simulink model "MATE_SynchronousMachine"  (R2024b)
settings: Solver=FixedStepDiscrete  StartTime=0.0  StopTime=6  FixedStep=Ts  RelTol=1e-4  EnableMultiTasking=on
PostLoadFcn:
  | Ts=25e-6;offset=4;
InitFcn:
  | Ts=25e-6;offset=4;
undefined symbols (not defined in the file): DiscIntNeverNeededParam, MATE, Phase, Rsnu, Single
libraries: fl_lib x79, nesl_utility x53, ee_lib x16, simetran x5, powerlib_extras x3, simulink_extras x2, simulink x2
(part 2 of 5)

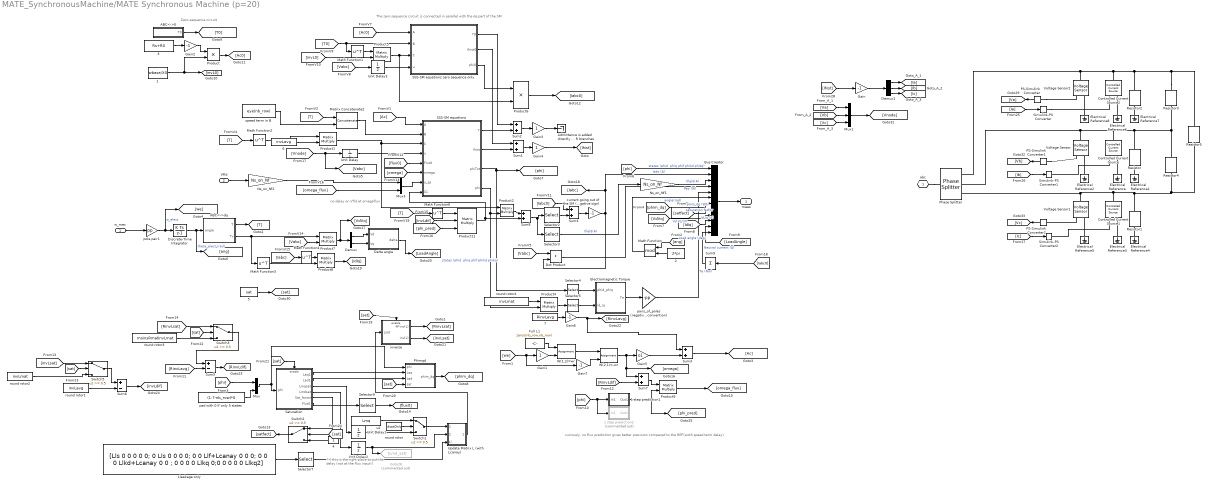
== system MATE_SynchronousMachine/MATE Synchronous Machine (p=20) ==
  note: ^
      | |
      | this is the right place to put the delay
      | (not at the flux input!)
  note: Zero-sequence circuit
  note: The zero sequence circuit is connected in parallel with the dq part of the SM
  note: curiously, no flux prediction gives better precision compared to the REF(woth speed term delay)
  note: no delay on Vfld et omegaflux
  "   w_mec" : Inport
  "   Vfld" : Inport  Port=2
  1 : Constant  Value=wbase/X0
  1 step prediction1 : Subsystem
  1 step prediction2 : Subsystem  Commented=on
  2 : Constant  Value=2*pi
  3 : Constant  Value=Rs+R0
  4 : Constant
  5 : Constant  Value=sat
  6 : Constant  Value=invLavg
  7 : Constant  Value=RinvLavg
  ABC<->0 : Subsystem
  ABC<->dq : Subsystem
  Admittance is added directly with R branches : Terminator
  Bus Creator : BusCreator  Inputs=12
  Controlled Current Source : fl_lib/Electrical/Electrical Sources/Controlled Current Source
  Controlled Current Source1 : fl_lib/Electrical/Electrical Sources/Controlled Current Source
  Controlled Current Source2 : fl_lib/Electrical/Electrical Sources/Controlled Current Source
  Delta angle : Subsystem
  Demux : Demux  Outputs=2
  Demux1 : Demux  Outputs=3
      settings: DisplayOption=none
  Discrete-Time Integrator : DiscreteIntegrator  InitialCondition=theta_0  SampleTime=Ts  ICPrevOutput=DiscIntNeverNeededParam  ICPrevScaledInput=DiscIntNeverNeededParam
  Dot Product : DotProduct  OutDataTypeStr=Inherit: Inherit via internal rule
  Electrical Reference{,1..8} (9 alike) : fl_lib/Electrical/Electrical Elements/Electrical Reference
  Electromagnetic Torque : Subsystem
  Full L1 : Constant  Value=zeros(nb_row,nb_row)
  Gain : Gain  Gain=-1
  Gain1 : Gain  SaturateOnIntegerOverflow=on  OutDataTypeStr=Inherit: Same as input  ParamDataTypeStr=Inherit: Same as input
  Gain2 : Gain  Gain=-1
  Gain3 : Gain
  Gain4 : Gain
  Gain5 : Gain  Gain=o1
  Gain6 : Gain  Gain=-1
  Gain7 : Gain  Gain=-1  SaturateOnIntegerOverflow=on  OutDataTypeStr=Inherit: Same as input  ParamDataTypeStr=Inherit: Same as input
  Goto28 : Goto  Commented=on  GotoTag=Lmd_sat
  Lleakage only : Constant  Value="[Lls 0 0 0 0 0; 0 Lls 0 0  0 0; 0 0 Llf+Lcanay 0 0 0; 0 0 0 Llkd+Lcanay 0 0 ; 0 0 0 0 Llkq 0;0 0 0 0 0 Llkq2]"
  Math Function : Math  Operator=mod  SignedPower=on
  Math Function{1..4,6} (5 alike) : Math  Operator=transpose  SignedPower=on
  Matrix Concatenate2 : Concatenate  Mode=Multidimensional array  ConcatenateDimension=2
  Mux : Mux  Inputs=2
  Mux1 : Mux  Inputs=3
  Mux3 : Mux  Inputs=2
  Ns_on_Nf1 : Gain  Gain=Ns_on_Nf
  Ns_on_Nf2 : Gain  Gain=Ns_on_Nf
  PS-Simulink Converter : nesl_utility/PS-Simulink Converter  PhysicalDomain=network_engine_domain  SubClassName=ps_output  LeftPortType=input  RightPortType=output  PseudoPeriodic=off  Frequencies=[]  VectorFormat=inherit  Unit=inherit  AffineConversion=off
  PS-Simulink Converter1 : nesl_utility/PS-Simulink Converter  PhysicalDomain=network_engine_domain  SubClassName=ps_output  LeftPortType=input  RightPortType=output  PseudoPeriodic=off  Frequencies=[]  VectorFormat=inherit  Unit=inherit  AffineConversion=off
  PS-Simulink Converter2 : nesl_utility/PS-Simulink Converter  PhysicalDomain=network_engine_domain  SubClassName=ps_output  LeftPortType=input  RightPortType=output  PseudoPeriodic=off  Frequencies=[]  VectorFormat=inherit  Unit=inherit  AffineConversion=off
  Phase Splitter : ee_lib/Connectors & References/Phase Splitter
  Phimqd : Subsystem
  Product : Product  RndMeth=Zero
  Product{1..2,4..5,7..9} (7 alike) : Product  Multiplication=Matrix(*)  SaturateOnIntegerOverflow=on  OutDataTypeStr=Inherit: Same as first input
  Product11 : Product  Inputs=3  Multiplication=Matrix(*)  SaturateOnIntegerOverflow=on  OutDataTypeStr=Inherit: Same as first input
  Product6 : Product  SaturateOnIntegerOverflow=on  OutDataTypeStr=Inherit: Same as first input
  Resistor : fl_lib/Electrical/Electrical Elements/Resistor  R=ResistanceM(2,2) Ohm  i_specify=off  i_priority=None  i=0 A  i_nominal_specify=off  i_nominal_value=1  i_nominal_unit=A  v_specify=off  v_priority=None  v=0 V  v_nominal_specify=off  v_nominal_value=1  v_nominal_unit=V
  Resistor1 : fl_lib/Electrical/Electrical Elements/Resistor  R=ResistanceM(3,3) Ohm  i_specify=off  i_priority=None  i=0 A  i_nominal_specify=off  i_nominal_value=1  i_nominal_unit=A  v_specify=off  v_priority=None  v=0 V  v_nominal_specify=off  v_nominal_value=1  v_nominal_unit=V
  Resistor2 : fl_lib/Electrical/Electrical Elements/Resistor  R=ResistanceM(1,1) Ohm  i_specify=off  i_priority=None  i=0 A  i_nominal_specify=off  i_nominal_value=1  i_nominal_unit=A  v_specify=off  v_priority=None  v=0 V  v_nominal_specify=off  v_nominal_value=1  v_nominal_unit=V
  Resistor3 : fl_lib/Electrical/Electrical Elements/Resistor  R=ResistanceM(1,2) Ohm  i_specify=off  i_priority=None  i=0 A  i_nominal_specify=off  i_nominal_value=1  i_nominal_unit=A  v_specify=off  v_priority=None  v=0 V  v_nominal_specify=off  v_nominal_value=1  v_nominal_unit=V
  Resistor4 : fl_lib/Electrical/Electrical Elements/Resistor  R=ResistanceM(2,3) Ohm  i_specify=off  i_priority=None  i=0 A  i_nominal_specify=off  i_nominal_value=1  i_nominal_unit=A  v_specify=off  v_priority=None  v=0 V  v_nominal_specify=off  v_nominal_value=1  v_nominal_unit=V
  Resistor5 : fl_lib/Electrical/Electrical Elements/Resistor  R=ResistanceM(1,3) Ohm  i_specify=off  i_priority=None  i=0 A  i_nominal_specify=off  i_nominal_value=1  i_nominal_unit=A  v_specify=off  v_priority=None  v=0 V  v_nominal_specify=off  v_nominal_value=1  v_nominal_unit=V
  SSS-SM equations : Subsystem
  SSS-SM equations zero sequence only : Subsystem
  Saturation : Subsystem
  Selector2 : Selector  InputPortWidth=4  IndexOptions=Index vector (dialog)  Indices=[1 2 3 ]  OutputSizes=1
  Selector3 : Selector  InputPortWidth=4  IndexOptions=Index vector (dialog)  Indices=[4 ]  OutputSizes=1
  Selector4 : Selector  InputPortWidth=nb_row  IndexOptions=Index vector (dialog)  Indices=[1 2]  OutputSizes=1
  Selector5 : Selector  InputPortWidth=nb_row  IndexOptions=Index vector (dialog)  Indices=[1 2]  OutputSizes=1
  Selector7 : Selector  NumberOfDimensions=2  InputPortWidth=3  IndexOptions=Index vector (dialog),Index vector (dialog)  Indices=[1:nb_row],[1:nb_row]  OutputSizes=1,1
  Selector9 : Selector  InputPortWidth=6  IndexOptions=Index vector (dialog)  Indices=[1:nb_row]  OutputSizes=1
  Simulink-PS Converter : nesl_utility/Simulink-PS Converter  PhysicalDomain=network_engine_domain  SubClassName=ps_input  LeftPortType=input  RightPortType=output  PseudoPeriodic=off  Frequencies=[]  NoiseDistribution=none  NoiseParameters=[]  Unit=1  AffineConversion=off  FilteringAndDerivatives=provide  SimscapeFilterOrder=1  InputFilterTimeConstant=0.001  UdotUserProvided=0
  Simulink-PS Converter1 : nesl_utility/Simulink-PS Converter  PhysicalDomain=network_engine_domain  SubClassName=ps_input  LeftPortType=input  RightPortType=output  PseudoPeriodic=off  Frequencies=[]  NoiseDistribution=none  NoiseParameters=[]  Unit=1  AffineConversion=off  FilteringAndDerivatives=provide  SimscapeFilterOrder=1  InputFilterTimeConstant=0.001  UdotUserProvided=0
  Simulink-PS Converter2 : nesl_utility/Simulink-PS Converter  PhysicalDomain=network_engine_domain  SubClassName=ps_input  LeftPortType=input  RightPortType=output  PseudoPeriodic=off  Frequencies=[]  NoiseDistribution=none  NoiseParameters=[]  Unit=1  AffineConversion=off  FilteringAndDerivatives=provide  SimscapeFilterOrder=1  InputFilterTimeConstant=0.001  UdotUserProvided=0
  Sum{1..4,7..8} (6 alike) : Sum  SaturateOnIntegerOverflow=on
  Sum5 : Sum  Inputs=+-  SaturateOnIntegerOverflow=on
  Sum6 : Sum  Inputs=+-  SaturateOnIntegerOverflow=on
  Sum9 : Sum  Inputs=+  SaturateOnIntegerOverflow=on
  Switch{1..3,5} (4 alike) : Switch  Threshold=0.5  SaturateOnIntegerOverflow=off  InputSameDT=off
  Unit Delay : UnitDelay  SampleTime=Ts  HasFrameUpgradeWarning=on
  Unit Delay1 : UnitDelay  InitialCondition=Lmq  SampleTime=Ts  HasFrameUpgradeWarning=on
  Unit Delay2 : UnitDelay  InitialCondition=Lmd  SampleTime=Ts  HasFrameUpgradeWarning=on
  Unit Delay3 : UnitDelay  SampleTime=Ts  HasFrameUpgradeWarning=on
  Update Matrix L (with Lcanay) : Subsystem
  Voltage Sensor : fl_lib/Electrical/Electrical Sensors/Voltage Sensor
  Voltage Sensor1 : fl_lib/Electrical/Electrical Sensors/Voltage Sensor
  Voltage Sensor2 : fl_lib/Electrical/Electrical Sensors/Voltage Sensor
  W(1,2)=wr : Assignment  NumberOfDimensions=2  IndexOptions=Index vector (dialog),Index vector (dialog)  Indices=1,2  OutputSizes=1,1
  W(2,1)=-wr : Assignment  NumberOfDimensions=2  IndexOptions=Index vector (dialog),Index vector (dialog)  Indices=2,1  OutputSizes=1,1
  current going out of the SM (negative sign) : Gain  Gain=-1
  inverse : Subsystem
  pad with 0 if only 5 states : Constant  Value=(1:7-nb_row)*0
  pairs_of_poles (negative sign for generator convention) : Gain  Gain=-pp
  pole pair1 : Gain  Gain=pp
  round rotor : Constant  Value=dsatOnly
  round rotor1 : Constant  Value=invLavg
  round rotor2 : Constant  Value=invLmat
  round rotor3 : Constant  Value=moinsRmatinvLmat
  round rotor4 : Constant  Value=invLmat
  speed term in B : Constant  Value=eye(nb_row)  VectorParams1D=off
  u2 : Constant  Value=Lmq
  "abc   " : PMIOPort  Side=Right
  "meas   " : Outport
  wires:
  Mux3/1 -> SSS-SM equations/7(u_sp)
  1 step prediction1/1(Out1) -> Product9/2, [phi_pred]
  [sat] -> Switch2/2
  Switch5/1 -> Sum6/1
  [sat] -> Switch5/2
  [sat] -> Switch3/2
  [sat] -> Saturation/Enable
  [sat] -> Phimqd/4(sat)
  [sat] -> inverse/Enable
  5/1 -> [sat]
  [invLsat] -> Switch5/1
  round rotor2/1 -> Switch5/3
  inverse/2(inv(L)) -> [invLsat]
  Gain3/1 -> Admittance is added directly with R branches/1
  "   Vfld"/1 -> Ns_on_Nf2/1
  Ns_on_Nf2/1 -> Mux3/1
  Switch3/1 -> Sum5/1
  [RinvLsat] -> Switch3/1
  round rotor3/1 -> Switch3/3
  inverse/1(-R*inv(L)) -> [RinvLsat]
  Update Matrix L (with Lcanay)/1(Lsat) -> inverse/1(Lsat)
  Sum9/1 -> Bus Creator/12  "Neutral current (A)"
  [Iabc0] -> Sum9/1
  [Vnode] -> Unit Delay/1, [Vabc]
  SSS-SM equations zero sequence only/2(Ihist0) -> Sum1/1
  SSS-SM equations zero sequence only/1(Y0) -> Sum2/1
  [phi] -> 1 step prediction2/1(In1), 1 step prediction1/1(In1)
  [omega_flux] -> Mux3/2
  round rotor4/1 -> Product4/1
  Product11/1 -> Sum8/2, SSS-SM equations/8(C1)
  Sum8/1 -> Selector2/1, Selector3/1
  Product2/1 -> Sum8/1
  [Iabc0] -> Sum4/1
  [phi_pred] -> Product11/3
  [invLdif] -> Product11/2
  Math Function6/1 -> Product11/1
  [T] -> Math Function6/1
  Sum6/1 -> [invLdif]
  round rotor1/1 -> Sum6/2
  6/1 -> Product1/2
  Sum7/1 -> Product9/1
  [RinvLdif] -> Sum7/2
  Sum5/1 -> [RinvLdif]
  Gain6/1 -> [RinvLavg], Sum3/1
  [RinvLavg] -> Sum5/2
  7/1 -> Gain6/1
  Ns_on_Nf1/1 -> Bus Creator/3  "Ifield(A)"
  Product9/1 -> [omega_flux]
  Bus Creator/1 -> "meas   "/1
  Matrix Concatenate2/1 -> SSS-SM equations/2(B)
  speed term in B/1 -> Matrix Concatenate2/2
  [T] -> Matrix Concatenate2/1
  Gain5/1 -> Sum3/2
  ABC<->dq/2(Tv) -> Product7/1, Math Function3/1
  [LoadAngle] -> Bus Creator/11  "Load angle (deg)"
  [IdIq] -> Bus Creator/10  "Id Iq (A)"
  [VdVq] -> Bus Creator/9  "Vd Vq (V)"
  Math Function4/1 -> Product8/1
  Math Function3/1 -> Product8/2
  [Iabc] -> Math Function4/1
  Product8/1 -> [IdIq]
  Delta angle/1(delta) -> [LoadAngle]
  [Vabc] -> Product7/2
  Demux/1 -> Delta angle/1(Vd)
  Demux/2 -> Delta angle/2(Vq)
  Product7/1 -> Demux/1, [VdVq]
  pole pair1/1 -> [we], Discrete-Time Integrator/1  "w_elect"
  ABC<->dq/1(T) -> [T]
  Discrete-Time Integrator/1 -> ABC<->dq/1(angle), [ang]  "theta_elect (rad)"
  SSS-SM equations/3(phiTot) -> [phi], Selector4/1  "states (phid  phiq phif phikd phikq)"
  Unit Delay/1 -> SSS-SM equations/4(u)
  Gain7/1 -> W(2,1)=-wr/2
  W(1,2)=wr/1 -> W(2,1)=-wr/1
  [we] -> Gain1/1, Gain7/1
  [T] -> Math Function2/1
  Product1/1 -> Product2/1, SSS-SM equations/3(C)
  Math Function2/1 -> Product1/1
  Gain1/1 -> W(1,2)=wr/2
  Selector3/1 -> Ns_on_Nf1/1  "Ifield(A)"
  Electromagnetic Torque/1(Te) -> pairs_of_poles (negative sign for generator convention)/1
  Selector5/1 -> Electromagnetic Torque/2(id_iq)
  Selector4/1 -> Electromagnetic Torque/1(phid_phiq)
  Product4/1 -> Selector5/1
  pairs_of_poles (negative sign for generator convention)/1 -> Bus Creator/5  "Te (Nm)"
  [Vabc] -> Dot Product/1
  Dot Product/1 -> Bus Creator/4  "Peo (W)"
  current going out of the SM (negative sign)/1 -> [Iabc], Bus Creator/2, Dot Product/2  "Iabc (A)"
  "   w_mec"/1 -> pole pair1/1
  [ang] -> Math Function/1
  Math Function/1 -> Bus Creator/6  "angle(rad)"
  2/1 -> Math Function/2
  [phi] -> Mux/1
  Saturation/1(Laq1) -> Phimqd/2(Laq)
  Saturation/2(Lad1) -> Phimqd/3(Lad)
  Saturation/3(Lmqsat) -> Unit Delay1/1
  Saturation/4(Lmdsat) -> Unit Delay2/1
  Switch1/1 -> Update Matrix L (with Lcanay)/1(Lmq)
  round rotor/1 -> Switch1/2
  Unit Delay2/1 -> Goto28/1, Update Matrix L (with Lcanay)/2(Lmd)
  Lleakage only/1 -> Selector7/1
  [phim_dq] -> Bus Creator/7  "phim_dq (Wb)"
  Phimqd/1(phim_dq) -> [phim_dq]
  Unit Delay1/1 -> Switch1/3
  u2/1 -> Switch1/1
  Selector7/1 -> Update Matrix L (with Lcanay)/3(Ll)
  [Ac] -> SSS-SM equations/1(A)
  pad with 0 if only 5 states/1 -> Mux/2
  Mux/1 -> Saturation/1(phi), Phimqd/1(phi)
  ABC<->0/1(T0) -> [T0]
  3/1 -> Gain2/1
  Gain2/1 -> Product/1
  1/1 -> [invL0], Product/2
  Product/1 -> [Ac0]
  [Ac0] -> SSS-SM equations zero sequence only/1(A)
  [Vabc] -> Unit Delay3/1
  Unit Delay3/1 -> SSS-SM equations zero sequence only/4(u)
  [T0] -> Math Function1/1, SSS-SM equations zero sequence only/2(B)
  Math Function1/1 -> Product5/1
  [invL0] -> Product5/2
  Product5/1 -> Product6/2, SSS-SM equations zero sequence only/3(C)
  Sum1/1 -> Gain4/1
  SSS-SM equations/2(Ihist) -> Sum1/2
  SSS-SM equations/1(Y) -> Sum2/2
  Sum2/1 -> Gain3/1
  Selector2/1 -> Sum4/2
  Sum4/1 -> current going out of the SM (negative sign)/1
  [satfact] -> Bus Creator/8  "saturation factor"
  Switch2/1 -> [satfact]
  Saturation/5(Sat_factor) -> Switch2/1
  4/1 -> Switch2/3
  Saturation/6(Flux0) -> Selector9/1
  [flux0] -> SSS-SM equations/5(Flux0)
  W(2,1)=-wr/1 -> [omega], Sum7/1, Gain5/1
  Sum3/1 -> [Ac]
  Full L1/1 -> W(1,2)=wr/1
  [omega] -> SSS-SM equations/6(omega)
  [phi] -> Bus Creator/1  "states (phid  phiq phif phikd phikq)"
  Selector9/1 -> [flux0]
  SSS-SM equations/4(phi) -> Product2/2, Product4/2
  PS-Simulink Converter1/1 -> [Vb]
  Mux1/1 -> [Vnode]
  Demux1/2 -> [Ib]
  Demux1/1 -> [Ia]
  [Vc] -> Mux1/3
  Gain/1 -> Demux1/1
  PS-Simulink Converter/1 -> [Va]
  [Ic] -> Simulink-PS Converter2/1
  Demux1/3 -> [Ic]
  [Va] -> Mux1/1
  [Ihist] -> Gain/1
  [Vb] -> Mux1/2
  PS-Simulink Converter2/1 -> [Vc]
  [Ib] -> Simulink-PS Converter1/1
  [Ia] -> Simulink-PS Converter/1
  Gain4/1 -> [Ihist]
  SSS-SM equations zero sequence only/3(phi0) -> Product6/1
  Product6/1 -> [Iabc0]
  connections:
  Controlled Current Source/LConn1 -- Resistor4/LConn1 -- Resistor3/RConn1 -- Resistor/LConn1 -- Phase Splitter/RConn2 -- Voltage Sensor/LConn1
  Resistor4/RConn1 -- Resistor5/RConn1 -- Controlled Current Source1/LConn1 -- Phase Splitter/RConn3 -- Voltage Sensor1/LConn1 -- Resistor1/LConn1
  Resistor3/LConn1 -- Resistor5/LConn1 -- Resistor2/LConn1 -- Controlled Current Source2/LConn1 -- Phase Splitter/RConn1 -- Voltage Sensor2/LConn1
  Electrical Reference2/LConn1 -- Voltage Sensor/RConn2
  Electrical Reference3/LConn1 -- Controlled Current Source1/RConn2
  Electrical Reference1/LConn1 -- Resistor/RConn1
  Electrical Reference7/LConn1 -- Resistor2/RConn1
  Controlled Current Source1/RConn1 -- Simulink-PS Converter2/RConn1
  "abc   "/RConn1 -- Phase Splitter/LConn1
  Electrical Reference4/LConn1 -- Resistor1/RConn1
  Electrical Reference6/LConn1 -- Controlled Current Source2/RConn2
  PS-Simulink Converter1/LConn1 -- Voltage Sensor/RConn1
  Simulink-PS Converter/RConn1 -- Controlled Current Source2/RConn1
  Electrical Reference/LConn1 -- Controlled Current Source/RConn2
  Voltage Sensor1/RConn1 -- PS-Simulink Converter2/LConn1
  Controlled Current Source/RConn1 -- Simulink-PS Converter1/RConn1
  PS-Simulink Converter/LConn1 -- Voltage Sensor2/RConn1
  Electrical Reference8/LConn1 -- Voltage Sensor2/RConn2
  Electrical Reference5/LConn1 -- Voltage Sensor1/RConn2

== system MATE_SynchronousMachine/MATE_LineCommutatedConverter ==
  g : Inport
  MATEPREP : Subsystem  Commented=on
  MATE_AGGREG : Subsystem
  Phase Splitter2 : ee_lib/Connectors & References/Phase Splitter
  abc : PMIOPort  Side=Left
  + : PMIOPort  Port=2  Side=Right
  - : PMIOPort  Port=3  Side=Right
  meas : Outport
  wires:
  g/1 -> MATEPREP/1(g), MATE_AGGREG/1(g)
  MATE_AGGREG/1(meas) -> meas/1
  connections:
  MATEPREP/RConn2 -- MATE_AGGREG/RConn2 -- -/RConn1
  MATEPREP/RConn1 -- MATE_AGGREG/RConn1 -- +/RConn1
  Phase Splitter2/RConn1 -- MATEPREP/LConn1 -- MATE_AGGREG/LConn1
  Phase Splitter2/RConn2 -- MATEPREP/LConn2 -- MATE_AGGREG/LConn2
  Phase Splitter2/RConn3 -- MATEPREP/LConn3 -- MATE_AGGREG/LConn3
  abc/RConn1 -- Phase Splitter2/LConn1

== system MATE_SynchronousMachine/Mesure et visualisation ==
  Discrete Mean value : Subsystem  mask(Discrete Mean value){Freq=60, Vinit=0, Ts=Ts}
      mask prompts: Freq "Fundamental frequency (Hz):"; Vinit "Initial input (DC component):"; Ts "Sample time:"
      mask help: Compute the mean value of the input signal over a running window of one cycle of the specified fundamental frequency.
      mask init:
      | SamplesPerCycle=1/Freq/Ts;
      | RoundSamplesPerCycle=ceil(SamplesPerCycle);
      | Delay=RoundSamplesPerCycle*Ts;
      | Corr1=(SamplesPerCycle-RoundSamplesPerCycle)/2;
      | Corr2=(SamplesPerCycle-RoundSamplesPerCycle)/SamplesPerCycle;
      | K1=Corr1*Corr2;
      | K2=Corr2 + Corr1*Corr2;
      mask Display: disp('Mean\n(discrete)')
  Mux : Mux  Inputs=2
  Mux3 : Mux  Inputs=2
  Mux4 : Mux  Inputs=2
  V1 Vref : Outport
  If IIfref : Outport  Port=2
  Vcc : Outport  Port=3
  wires:
  Discrete Mean value/1(Mean) -> Mux/2
  [Ucc] -> Mux/1, Discrete Mean value/1(In)
  Mux/1 -> Vcc/1  "Vcc - Vcc moyen (V)"
  [If] -> Mux3/1
  [Ifref] -> Mux3/2
  Mux3/1 -> If IIfref/1
  [V1] -> Mux4/1
  [Vref] -> Mux4/2
  Mux4/1 -> V1 Vref/1

== system MATE_SynchronousMachine/Model Initialization ==

== system MATE_SynchronousMachine/PQ ==
  note: 1) P = Va*Ia + Vb*Ib + Vc*Ic
  note: 2) Q = 1/sqrt(3)* (Vbc*Ia + Vca*Ib + Vab*Ic)
  note: This block computes the 3-phase instantaneous real power and reactive power using the following equations:
  note: Note: Equation 2 is valid only for a balanced and harmonic-free system.
  Vabc : Inport  PortDimensions=3
  Iabc : Inport  Port=2  PortDimensions=3
  Demux : Demux  Outputs=3
      settings: DisplayOption=none
  Mux : Mux  Inputs=3
  Mux1 : Mux  Inputs=2
  Product1 : Product  InputSameDT=on  SaturateOnIntegerOverflow=on  OutDataTypeStr=Inherit: Same as first input
  Product3 : Product  InputSameDT=on  SaturateOnIntegerOverflow=on  OutDataTypeStr=Inherit: Same as first input
  Sum : Sum  Inputs=+-  InputSameDT=on  SaturateOnIntegerOverflow=on  OutDataTypeStr=Inherit: Same as first input
  Sum1 : Sum  Inputs=1  InputSameDT=on  SaturateOnIntegerOverflow=on  OutDataTypeStr=Inherit: Same as first input
  Sum4 : Sum  Inputs=1  InputSameDT=on  SaturateOnIntegerOverflow=on  OutDataTypeStr=Inherit: Same as first input
  Sum5 : Sum  Inputs=+-  InputSameDT=on  SaturateOnIntegerOverflow=on  OutDataTypeStr=Inherit: Same as first input
  Sum6 : Sum  Inputs=+-  InputSameDT=on  SaturateOnIntegerOverflow=on  OutDataTypeStr=Inherit: Same as first input
  pu->V : Gain  Gain=1/sqrt(3)  SaturateOnIntegerOverflow=on  OutDataTypeStr=Inherit: Same as input  ParamDataTypeStr=Inherit: Same as input
  PQ : Outport  VectorParamsAs1DForOutWhenUnconnected=off
  wires:
  Sum1/1 -> pu->V/1
  Product3/1 -> Sum1/1
  Product1/1 -> Sum4/1
  Vabc/1 -> Product1/1, Demux/1
  Iabc/1 -> Product1/2, Product3/2
  Sum4/1 -> Mux1/1  "P"
  Demux/1 -> Sum/1, Sum6/2
  Demux/2 -> Sum/2, Sum5/1
  Demux/3 -> Sum5/2, Sum6/1
  Sum/1 -> Mux/3
  Sum5/1 -> Mux/1
  Sum6/1 -> Mux/2
  Mux/1 -> Product3/1
  pu->V/1 -> Mux1/2  "Q"
  Mux1/1 -> PQ/1

== system MATE_SynchronousMachine/VI meas ==
  Kv2 : Gain  Gain=Kv  SaturateOnIntegerOverflow=on  OutDataTypeStr=Inherit: Same as input  ParamDataTypeStr=Inherit: Same as input
  Kv3 : Gain  Gain=Ki  SaturateOnIntegerOverflow=on  OutDataTypeStr=Inherit: Same as input  ParamDataTypeStr=Inherit: Same as input
  Meas : ee_lib/Sensors & Transducers/Current and Voltage Sensor (Three-Phase)  vMeasurementType=ee.enum.vmeasurement.lg  outputUnit=ee.enum.unit.si  SRated=100e6 A*V  VRated=24e3 V  I_specify=off  I_priority=None  I=[0, 0, 0] A  I_nominal_specify=off  I_nominal_value=1  I_nominal_unit=A  V_specify=off  V_priority=None  V=[0, 0, 0] V  V_nominal_specify=off  V_nominal_value=1  V_nominal_unit=V
      settings: InternalSimscapePortConfiguration="{\"Bottom\":[],\"Left\":[{\"id\":\"N1\",\"label\":\"~1\",\"type\":\"foundation.electrical.three_phase\"}],\"Right\":[{\"id\":\"V_output\",\"label\":\"V\",\"type\":\"output\"},{\"id\":\"I_output\",\"label\":\"I\",\"type\":\"output\"},{\"id\":\"N2\",\"label\":\"~2\",\"type\":\"foundation.electrical.three_phase\"}],\"Top\":[]}"
  PS-Simulink Converter : nesl_utility/PS-Simulink Converter  PhysicalDomain=network_engine_domain  SubClassName=ps_output  LeftPortType=input  RightPortType=output  PseudoPeriodic=off  Frequencies=[]  VectorFormat=inherit  Unit=inherit  AffineConversion=off
  PS-Simulink Converter1 : nesl_utility/PS-Simulink Converter  PhysicalDomain=network_engine_domain  SubClassName=ps_output  LeftPortType=input  RightPortType=output  PseudoPeriodic=off  Frequencies=[]  VectorFormat=inherit  Unit=inherit  AffineConversion=off
  + : PMIOPort  Side=Left
  - : PMIOPort  Port=2  Side=Right
  tag scope: IabcB13_8=global, VabcB13_8=global
  wires:
  Kv3/1 -> [IabcB13_8]
  Kv2/1 -> [VabcB13_8]
  PS-Simulink Converter1/1 -> Kv3/1
  PS-Simulink Converter/1 -> Kv2/1
  connections:
  Meas/RConn1 -- PS-Simulink Converter/LConn1
  Meas/LConn1 -- +/RConn1
  Meas/RConn2 -- PS-Simulink Converter1/LConn1
  Meas/RConn3 -- -/RConn1

== system MATE_SynchronousMachine/VI meas1 ==
  Kv2 : Gain  Gain=Kv  SaturateOnIntegerOverflow=on  OutDataTypeStr=Inherit: Same as input  ParamDataTypeStr=Inherit: Same as input
  Kv3 : Gain  Gain=Ki  SaturateOnIntegerOverflow=on  OutDataTypeStr=Inherit: Same as input  ParamDataTypeStr=Inherit: Same as input
  Meas : ee_lib/Sensors & Transducers/Current and Voltage Sensor (Three-Phase)  vMeasurementType=ee.enum.vmeasurement.lg  outputUnit=ee.enum.unit.si  SRated=100e6 A*V  VRated=24e3 V  I_specify=off  I_priority=None  I=[0, 0, 0] A  I_nominal_specify=off  I_nominal_value=1  I_nominal_unit=A  V_specify=off  V_priority=None  V=[0, 0, 0] V  V_nominal_specify=off  V_nominal_value=1  V_nominal_unit=V
      settings: InternalSimscapePortConfiguration="{\"Bottom\":[],\"Left\":[{\"id\":\"N1\",\"label\":\"~1\",\"type\":\"foundation.electrical.three_phase\"}],\"Right\":[{\"id\":\"V_output\",\"label\":\"V\",\"type\":\"output\"},{\"id\":\"I_output\",\"label\":\"I\",\"type\":\"output\"},{\"id\":\"N2\",\"label\":\"~2\",\"type\":\"foundation.electrical.three_phase\"}],\"Top\":[]}"
  PS-Simulink Converter : nesl_utility/PS-Simulink Converter  PhysicalDomain=network_engine_domain  SubClassName=ps_output  LeftPortType=input  RightPortType=output  PseudoPeriodic=off  Frequencies=[]  VectorFormat=inherit  Unit=inherit  AffineConversion=off
  PS-Simulink Converter1 : nesl_utility/PS-Simulink Converter  PhysicalDomain=network_engine_domain  SubClassName=ps_output  LeftPortType=input  RightPortType=output  PseudoPeriodic=off  Frequencies=[]  VectorFormat=inherit  Unit=inherit  AffineConversion=off
  + : PMIOPort  Side=Left
  - : PMIOPort  Port=2  Side=Right
  tag scope: Ifault=global, Vfault=global
  wires:
  PS-Simulink Converter/1 -> Kv2/1
  PS-Simulink Converter1/1 -> Kv3/1
  Kv2/1 -> [Vfault]
  Kv3/1 -> [Ifault]
  connections:
  Meas/RConn3 -- -/RConn1
  Meas/RConn2 -- PS-Simulink Converter1/LConn1
  Meas/LConn1 -- +/RConn1
  Meas/RConn1 -- PS-Simulink Converter/LConn1

== system MATE_SynchronousMachine/turbine1 ==
  feild : Inport
  Te : Inport  Port=2
  Peo : Inport  Port=3
  Gain : Gain  Gain=1/(2*pi*60/20)
  Gain1 : Gain  Gain=1/202e6
  Gain3 : Gain  Gain=202e6
  Gain4 : Gain  Gain=1/(2*pi*60/20)
  Hydraulic Turbine and Governor : Subsystem  mask(Hydraulic Turbine and Governor){sm=[ 10/3  0.07 ], gate=[  0.01  0.97518  -0.1  0.1 ], reg=[  0.05  1.163  0.105  0  0.01  ], hyd=[  0  2.67  ], dref=0, po=0.802}
      mask prompts: sm "Servo-motor [ Ka()  Ta(sec) ]:"; gate "Gate opening limits [ gmin,gmax(pu)    vgmin,vgmax(pu/s) ]:"; reg "Permanent droop and regulator  [ Rp() Kp() Ki() Kd() Td(s) ]:"; hyd "Hydraulic turbine [ beta()  Tw(sec) ]:"; dref "Droop reference (0=power error, 1=gate opening):"; po "Initial mechanical power (pu):"
      mask help: Implements a hydraulic turbine combined to a PID governor system.
      mask init:
      | %block = gcb;
      | %[Ts, WantBlockChoice,ka,ta,gmin,gmax,vgmin,vgmax,Rp,Kp,ki,kd,td,beta,tw,go] = powericon('HydraulicTurbineInit',block,sm,gate,reg,hyd,po);
      | ka =sm (1 ); 
      | ta =sm (2 ); 
      | gmin =gate (1 ); 
      | gmax =gate (2 ); 
      | vgmin =gate (3 ); 
      | vgmax =gate (4 ); 
      | Rp =reg (1 ); 
      | kp =reg (2 ); 
      | ki =reg (3 ); 
      | kd =reg (4 ); 
      | td =reg (5 ); 
      | beta =hyd (1 ); 
      | tw =hyd (2 ); 
      | go =po *(gmax -gmin ); 
      | %powericon('SetInternalModels','set',block,WantBlockChoice);
      settings: OpenFcn=sps_rtmsupport('OpenFcn',gcbh)
      mask Help: helpview(psbhelp);
      mask Display: disp('')
  Mechanical model : Subsystem  mask(Synchronous machine mechanical model){J=3.4111e+06, F=0, fo=60/20, Ts=Ts}
      mask prompts: J "Inertia (kg.m^2)"; F "Friction (N.n.s)"; fo "Initial mechanical frequency (Hz)"; Ts "Sample Time (s)"
      mask help:
      | This is the mechanical equation of a synchronous machine.
      |
      | all values in SI.
      | J: inertia
      | F:friction
      | Te: torque input from the SM
      | Pin: power from the turbine
      | wmec: mechanical speed of the SM.
      | delta_wm: speed deviation
  Pref : Constant  Value=0.8
  Product1 : Product
  Terminator : Terminator
  wref : Constant
  w : Outport
  wires:
  Hydraulic Turbine and Governor/2(gate) -> Terminator/1
  Hydraulic Turbine and Governor/1(Pm) -> Gain3/1
  Gain1/1 -> Hydraulic Turbine and Governor/4(Pe0)
  Gain/1 -> Hydraulic Turbine and Governor/3(we)
  wref/1 -> Hydraulic Turbine and Governor/1(wref)
  Mechanical model/2(delta_wm) -> Gain4/1
  Pref/1 -> Product1/2
  Product1/1 -> Hydraulic Turbine and Governor/2(Pref)
  Gain3/1 -> Mechanical model/2(Pin)
  Mechanical model/1(wmec) -> Gain/1, w/1
  Gain4/1 -> Hydraulic Turbine and Governor/5(dw)
  feild/1 -> Product1/1
  Te/1 -> Mechanical model/1(Te)
  Peo/1 -> Gain1/1

== system MATE_SynchronousMachine/Command/Regulateur de courant ==
  If (pu) : Inport
  If_ref : Inport  Port=2
  Discrete 1st-Order Filter : Subsystem  mask(Discrete 1st-Order Filter){FilterType=Lowpass, Tc=1e-3, Ts=Ts, Initialize=off, Vac_Init=[0, 0, 60], Vdc_Init=0, PlotResponse=off, param1=[1 500 0.1]}
      mask prompts: FilterType "Filter Type:"; Tc "Time constant (s):"; Ts "Sample time:"; Initialize "Initialize filter states"; Vac_Init "AC initial input: [ Mag  Phase(degrees)  Freq(Hz) ]"; Vdc_Init "DC Initial input:"; PlotResponse "Plot filter response"; param1 "Frequency range(Hz) : [Start  End  Inc.]"
      mask init:
      | switch FilterType
      | case 1, % Lowpass
      |     X=[0 1 2 3 4];
      |     Y=[-2 -2 -3 -4 -4];
      |     numc=1;
      |     denc=[Tc 1];
      | case 2,   % Highpass
      |     X=[0 1 2 3 4];
      |     Y=[-4 -4 -3 -2 -2];
      |     numc=[1 0];
      |     denc=[1 1/Tc];
      | end
      | %
      | [Ac,Bc,Cc,Dc]=tf2ss(numc,denc);
      | %
      | %  Conversion to discrete transfer function
      | nstates = size(Ac,1);
      | if Ts<=0
      |     message = 'The Sample time parameter must be greater than zero. Note that specifying inherited sample time (-1) does not work for this block';
      |     error(message);
      | end
      | invexp = inv(eye(nstates) - (Ts/2)*Ac);
      | Ad = invexp*(eye(nstates) + (Ts/2)*Ac);
      | Bd = invexp*Bc;
      | Cd = Cc*invexp*Ts;
      | Dd = Cc*invexp*Bc*(Ts/2) + Dc;
      | %
      | if Initialize==1  % Compute initial conditions on states
      |     u1=Vac_Init(1)*exp(j*Vac_Init(2)*pi/180);
      |     u2=Vdc_Init*exp(j*90*pi/180);
      |     u=u1+u2;
      |     u0=imag(u); % input at  t=0;
      |     I=eye(size(Ac));
      |     sI1=I*j*(2*pi*Vac_Init(3));
      |     sI2=I*j*0;
      |     x=inv(sI1-Ac)*Bc*u1 + inv(sI2-Ac)*Bc*u2;
      |     x0c=imag(x);
      |     x0d=(I-Ac*Ts/2)*x0c/Ts - Bc/2*u0;
      | else
      |     x0d=0;
      | end
      | 
      | %
      | if PlotResponse==1 % Plot frequency and step response
      | t=[0:Tc/1000:7*Tc];
      | f=param1(1):param1(3):param1(2);
      | w=2*pi*f;
      | switch FilterType
      | 	case 1, % Lowpass
      | 		Ystep=1 - exp(-t/Tc);
      | 		RepFreq=1./(1+Tc*j.*w);
      | 	case 2,   % Highpass
      | 		Ystep=exp(-t/Tc);
      | 		RepFreq=1./(1 + (1./(Tc*j.*w)));
      | end
      | %
      | Mag=abs(RepFreq);
      | Pha=angle(RepFreq)*180/pi;
      | %
      | figure(1)
      | subplot(2,1,1)
      | plot(f,Mag)
      | grid
      | title('Bode Diagram')
      | ylabel('Magnitude')
      | subplot(2,1,2)
      | plot(f,Pha)
      | ylabel('Phase (deg)')
      | xlabel('Frequency (Hz)')
      | grid
      | figure(2)
      | plot(t,Ystep)
      | grid
      | ylabel('Amplitude')
      | xlabel('Time (s)')
      | title('Step Response')
      | end
      mask TypeOptions FilterType: Lowpass | Highpass
      mask Display: plot(X,Y);
  Discrete PI Controller1 : Subsystem  mask(Discrete PI Controller){Kp=400, Ki=1000, Par_Limits=[150 10], Init=79, Ts=Ts}
      mask prompts: Kp "Proportional gain (Kp):"; Ki "Integral gain (Ki):"; Par_Limits "Output limits: [ Upper   Lower ]"; Init "Output initial value:"; Ts "Sample time:"
      mask help: This block implements a basic discrete PI controller.
      mask init:
      | UpperLimit=Par_Limits(1);
      | LowerLimit=Par_Limits(2);
      mask Display: disp('PI');
  Sum : Sum  Inputs=|+-
  alpha : Outport
  wires:
  Discrete 1st-Order Filter/1(Out) -> Sum/1
  If (pu)/1 -> Discrete 1st-Order Filter/1(In)
  If_ref/1 -> Sum/2
  Sum/1 -> Discrete PI Controller1/1(Error)
  Discrete PI Controller1/1(Out) -> alpha/1

== system MATE_SynchronousMachine/Command/Regulateur de tension (Mode automatique) ==
  note: Regulateur de tension
  Vabc (pu) : Inport
  Vref : Inport  Port=2
  Discrete PI Controller1 : Subsystem  mask(Discrete PI Controller){Kp=Kp_V, Ki=Ki_V, Par_Limits=[2.46 0.33], Init=1, Ts=Ts}
      mask prompts: Kp "Proportional gain (Kp):"; Ki "Integral gain (Ki):"; Par_Limits "Output limits: [ Upper   Lower ]"; Init "Output initial value:"; Ts "Sample time:"
      mask help: This block implements a basic discrete PI controller.
      mask init:
      | UpperLimit=Par_Limits(1);
      | LowerLimit=Par_Limits(2);
      mask Display: disp('PI');
  Discrete 3-phase Positive-Sequence Fundamental Value : Subsystem  mask(Discrete 3-phase Positive-sequence fundamental value){Freq=60, Par_Init=[0 0], Ts=Ts}
      mask prompts: Freq "Fundamental frequency (Hz):"; Par_Init "Initial input (positive component): [ Mag  Phase(degrees) ]"; Ts "Sample time:"
      mask help: Compute the positive-sequence component of the input signal at the given fundamental frequency. The input is set of three balanced or unbalanced signals which may contain harmonics.
      mask init:
      | SamplesPerCycle=1/Freq/Ts;
      | RoundSamplesPerCycle=round(SamplesPerCycle);
      | Delay=RoundSamplesPerCycle*Ts - Ts/2;
      | Correction=SamplesPerCycle/RoundSamplesPerCycle - 1;
      | Real_Init=Par_Init(1)*cos(pi/180*Par_Init(2));
      | Imag_Init=Par_Init(1)*sin(pi/180*Par_Init(2));
      mask Display: disp('')
  Sum : Sum  Inputs=|-+
  Terminator : Terminator
  Iref : Outport
  tag scope: V1=global, Vref=global
  wires:
  Discrete 3-phase Positive-Sequence Fundamental Value/2(Phase) -> Terminator/1
  Vabc (pu)/1 -> Discrete 3-phase Positive-Sequence Fundamental Value/1(abc)
  Discrete PI Controller1/1(Out) -> Iref/1
  Sum/1 -> Discrete PI Controller1/1(Error)
  Vref/1 -> Sum/2, [Vref]
  Discrete 3-phase Positive-Sequence Fundamental Value/1(Mag) -> Sum/1, [V1]

== system MATE_SynchronousMachine/Command/Synchro Generateur d'mpulsions  ==
  Vabc_138 (pu) : Inport
  alpha(deg) : Inport  Port=2
  Demux : Demux  Outputs=3
  Discrete 3-phase PLL : Subsystem  mask(Discrete 3-phase PLL){Fmin=45, Par_Init=[0 60], ParK=[ 180 3200 1 ], Ts=Ts, AGC=on}
      mask prompts: Fmin "Minimum frequency (Hz):"; Par_Init "Initial inputs:[ Phase(degrees)   Frequency(Hz) ]"; ParK "Regulator gains [ Kp  Ki  Kd ]"; Ts "Sample time:"; AGC "Enable Automatic Gain Control"
      mask help:
      | This Phase Locked Loop (PLL) system can be used  to synchronize on a set of variable frequency, three-phase sinusoidal signals. If the Automatic Gain Control is enabled, the input (phase error) of the PLL regulator is scaled according to the input signals magnitude.
      |
      | For optimal performance, the following settings are recommended:
      |   [ Kp Ki  Kd ] = [ 180  3200  1 ]
      |   "Enable Automatic Gain Control" checked
      |
      | Input 1: Vector containing the normalized three-phase signals [Va Vb Vc]
      | Output 1:  Measured frequency (Hz) = w/(2pi)
      | Output 2:  Ramp w.t varying between  0 and 2*pi,
      |      synchronized on zero crossings of the fundamental (positive-sequence) of phase A.
      | Output 3: Vector [sin(wt) cos(wt)]
      mask init:
      | Kp=ParK(1);
      | Ki=ParK(2);
      | if length(ParK)==2
      |     Kd=0;
      | else
      |     Kd=ParK(3);
      | end    
      | Phase_Init=Par_Init(1);
      | Finit=Par_Init(2);
      settings: OpenFcn=power_openblockproxy();
      mask Display: disp('')
  Discrete Synchronized 12-Pulse Generator : Subsystem  mask(Discrete synchronized 12-pulse generator){Delta=D1 (lagging), pwidth=20, Double_Pulse=on, Ts=Ts}
      mask prompts: Delta "Delta winding connection"; pwidth "Pulse width (degrees)"; Double_Pulse "Double pulsing"; Ts "Sample time"
      mask help:
      | Use this block to fire the 12 thyristors of a 12-pulse converter.
      | Outputs 1 and 2 are two vectors of 6 pulses (0-1) to be sent to the two 6-pulse half bridges connected respectively to the Wye(Y) and Delta (D1 or D11) connected windings of the YYD converter transformer.
      | Pulses are individually synchronized on the 6 commutation voltages and generated alpha degrees after the increasing zero-crossings of the commutation voltages. The D pulses are either lagging or leading the Y pulses by 30 degrees.
      |
      | Input 'alpha_deg' :  Alpha firing signal (degrees).
      | Inputs 'A,B,C' : Phase-to-ground synchronization voltages  measured at the  primary side of the converter transformer.
      | Input 'Freq' : Frequency of the synchronization voltages (use a constant or the Freq PLL output)
      | Input 'Block' allows  blocking of the pulses when the applied signal is non zero.
      |
      | When the 'Douple pulsing' option is checked, two pulses are sent to each thyristor: a 1st pulse when the alpha angle is reached, then a 2nd pulse 60 degrees later, when the next thyristor is fired.
      mask init:
      | if (Delta == 1)
      |     D1 = 1;
      | else
      |     D1 = 0;
      | end
      mask TypeOptions Delta: D1 (lagging) | D11 (leading)
      mask Display: plot(0,0,100,100,[80 62 62 47 47 30],[40 40 60 60 40 40]-5)
  Ground2 : Ground
  Terminator : Terminator
  Terminator1 : Terminator
  Terminator2 : Terminator
  P : Outport
  wires:
  Vabc_138 (pu)/1 -> Discrete 3-phase PLL/1(Vabc(pu)), Demux/1
  Ground2/1 -> Discrete Synchronized 12-Pulse Generator/6(Block)
  alpha(deg)/1 -> Discrete Synchronized 12-Pulse Generator/1(alpha_deg)
  Demux/1 -> Discrete Synchronized 12-Pulse Generator/2(A)
  Demux/2 -> Discrete Synchronized 12-Pulse Generator/3(B)
  Demux/3 -> Discrete Synchronized 12-Pulse Generator/4(C)
  Discrete 3-phase PLL/1(Freq) -> Discrete Synchronized 12-Pulse Generator/5(Freq)
  Discrete Synchronized 12-Pulse Generator/2(PD) -> P/1
  Discrete 3-phase PLL/2(wt) -> Terminator/1
  Discrete 3-phase PLL/3(Sin_Cos) -> Terminator1/1
  Discrete Synchronized 12-Pulse Generator/1(PY) -> Terminator2/1

== system MATE_SynchronousMachine/MATE Synchronous Machine (p=20)/1 step prediction1 ==
  In1 : Inport
  Gain2 : Gain  Gain=2
  Gain3 : Gain  Gain=-1
  Sum5 : Sum  SaturateOnIntegerOverflow=on
  Unit Delay1 : UnitDelay  SampleTime=Ts  HasFrameUpgradeWarning=on
  Out1 : Outport
  wires:
  Sum5/1 -> Out1/1
  In1/1 -> Unit Delay1/1, Gain2/1
  Gain3/1 -> Sum5/2
  Gain2/1 -> Sum5/1
  Unit Delay1/1 -> Gain3/1

== system MATE_SynchronousMachine/MATE Synchronous Machine (p=20)/1 step prediction2 ==
  In1 : Inport
  Gain2 : Gain  Gain=2
  Gain3 : Gain  Gain=-1
  Sum5 : Sum  SaturateOnIntegerOverflow=on
  Unit Delay1 : UnitDelay  SampleTime=Ts  HasFrameUpgradeWarning=on
  Out1 : Outport
  wires:
  Unit Delay1/1 -> Gain3/1
  Gain2/1 -> Sum5/1
  Gain3/1 -> Sum5/2
  In1/1 -> Gain2/1, Unit Delay1/1
  Sum5/1 -> Out1/1

== system MATE_SynchronousMachine/MATE Synchronous Machine (p=20)/ABC<->0 ==
  note: (homopolar transform)
  Constant2 : Constant  Value=[1 1 1]  VectorParams1D=off
  Gain4 : Gain  Gain=sqrt(1/3)
  T0 : Outport
  wires:
  Gain4/1 -> T0/1  "T"
  Constant2/1 -> Gain4/1

== system MATE_SynchronousMachine/MATE Synchronous Machine (p=20)/ABC<->dq ==
  note: (rotor dq transformation reference frame)
  note: The Feild turn ratio gain has been moved directly in the Vfeild et IFeild signals
  angle : Inport
  Constant1 : Constant  Value="[0  ;0 ]"  VectorParams1D=off
  Constant2 : Constant  Value=[1 -0.5 -0.5;0 sqrt(3)/2 -sqrt(3)/2]
  Constant3 : Constant  Value=[0 0 0 Ns_on_Nf*0+1; 0 0 0 0 ; 0 0 0 0; 0 0 0 0]  VectorParams1D=off
  Divide : Product  Multiplication=Matrix(*)
  Gain2 : Gain  Gain=-1
  Gain4 : Gain  Gain=sqrt(2/3)
  Matrix Concatenate : Concatenate  Mode=Multidimensional array  ConcatenateDimension=2
  Matrix Concatenate1 : Concatenate  Mode=Multidimensional array
  Mux6 : Mux
  Reshape4 : Reshape  OutputDimensionality=Customize  OutputDimensions=[2,2]
  Selector : Selector  NumberOfDimensions=2  InputPortWidth=3  IndexOptions=Index vector (dialog),Index vector (dialog)  Indices=[1:nb_row-2],[1:4]  OutputSizes=1,1
  Trigonometric Function1 : Trigonometry  Operator=cos
  Trigonometric Function2 : Trigonometry
  T : Outport
  Tv : Outport  Port=2
  wires:
  Gain4/1 -> Tv/1, Matrix Concatenate/1  "T"
  Trigonometric Function1/1 -> Mux6/1, Mux6/4
  Trigonometric Function2/1 -> Gain2/1, Mux6/3
  Mux6/1 -> Reshape4/1
  Reshape4/1 -> Divide/1
  Constant2/1 -> Divide/2
  Divide/1 -> Gain4/1
  Gain2/1 -> Mux6/2
  Constant1/1 -> Matrix Concatenate/2
  Matrix Concatenate/1 -> Matrix Concatenate1/1
  Constant3/1 -> Selector/1
  Matrix Concatenate1/1 -> T/1
  angle/1 -> Trigonometric Function1/1, Trigonometric Function2/1
  Selector/1 -> Matrix Concatenate1/2

== system MATE_SynchronousMachine/MATE Synchronous Machine (p=20)/Delta angle ==
  Vd : Inport  PortDimensions=1
  Vq : Inport  Port=2  PortDimensions=1
  Cartesian to Polar : Subsystem  mask(Cart2Polar){}
      mask help:
      | Transformation from cartesian to polar coordinates.
      | [x, y] -> [r, theta]
      |
      | r = sqrt(x^2 + y^2);
      | theta = atan(y/x);
      mask Help: Unmask this block for more help.
      mask Display: plot(0,0,100,100,[24,20,15,20,20],[85,95,85,95,20],[80,20,95,85,95,85],[70,20,20,15,20,24],[56,56,55,52,50,46],[20,26,31,35,38,42])
  Radians to Degrees : Subsystem  mask(RadiansToDegrees){}
      mask help:
      | Conversion from Radians to Degrees.
      |
      | D=180/pi*R
      mask Help: This block converts from Radians to Degrees.
      mask Display: disp('R2D')
  Terminator2 : Terminator
  delta : Outport
  wires:
  Vd/1 -> Cartesian to Polar/2(y)
  Radians to Degrees/1(Degrees out) -> delta/1  "delta"
  Vq/1 -> Cartesian to Polar/1(x)
  Cartesian to Polar/1(r) -> Terminator2/1
  Cartesian to Polar/2(theta) -> Radians to Degrees/1(Radians in)

== system MATE_SynchronousMachine/MATE Synchronous Machine (p=20)/Electromagnetic Torque ==
  note: Te computed from stator fluxes and currents
  note: Te=phids*Iqs - phiqs*Ids
  phid_phiq : Inport
  id_iq : Inport  Port=2
  1-2 : Gain  Gain=[1 -1]
  Dot Product : DotProduct  OutDataTypeStr=Inherit: Inherit via internal rule
  Selector2 : Selector  InputPortWidth=2  IndexOptions=Index vector (dialog)  Indices="[2  1]"  OutputSizes=1
  Te : Outport
  wires:
  id_iq/1 -> Selector2/1
  Selector2/1 -> Dot Product/2  "iqs ids"
  phid_phiq/1 -> 1-2/1  "phids phiqs"
  Dot Product/1 -> Te/1
  1-2/1 -> Dot Product/1

== system MATE_SynchronousMachine/MATE Synchronous Machine (p=20)/Phimqd ==
  note: phimq=  phiqs*(Laq/Ll)   +phikq1*(Laq/Llkq1)  +phikq2*(Laq/Llkq2)
      | phimd=  phids*(Lad/Ll)   +phifd*(Lad/Llfd)  + phikd*(Lad/Llkd)
  note: Laq
  note: Lad
  phi : Inport
  Laq : Inport  Port=2
  Lad : Inport  Port=3
  sat : Inport  Port=4
  1/Ll_d : Gain  Gain="[1/Lls   1/Llf 1/Llkd ]"  SaturateOnIntegerOverflow=on  OutDataTypeStr=Inherit: Same as input  ParamDataTypeStr=Inherit: Same as input
  1/Ll_q : Gain  Gain=[1/Lls 1/Llkq 1/Llkq2]  SaturateOnIntegerOverflow=on  OutDataTypeStr=Inherit: Same as input  ParamDataTypeStr=Inherit: Same as input
  Constant2 : Constant  Value=Lad
  Constant4 : Constant  Value=Laq
  Mux1 : Mux  Inputs=2
  Product1 : Product  RndMeth=Zero
  Product3 : Product  RndMeth=Zero
  Switch : Switch  Threshold=0.5  SaturateOnIntegerOverflow=off  InputSameDT=off
  Switch1 : Switch  Threshold=0.5  SaturateOnIntegerOverflow=off  InputSameDT=off
  "phid phifd phikd " : Selector  InputPortWidth=7  IndexOptions=Index vector (dialog)  Indices=[1 3 4]  OutputSizes=1
  phiq phikq1 (phikq2) : Selector  InputPortWidth=7  IndexOptions=Index vector (dialog)  Indices=[2 5 6]  OutputSizes=1
  sum : Sum  Inputs=+  InputSameDT=on  SaturateOnIntegerOverflow=on  OutDataTypeStr=Inherit: Same as first input
  sum1 : Sum  Inputs=+  InputSameDT=on  SaturateOnIntegerOverflow=on  OutDataTypeStr=Inherit: Same as first input
  phim_dq : Outport
  wires:
  Switch1/1 -> Product3/2
  Lad/1 -> Switch1/1
  Constant2/1 -> Switch1/3
  Laq/1 -> Switch/1
  Constant4/1 -> Switch/3
  sat/1 -> Switch/2, Switch1/2
  Switch/1 -> Product1/1
  sum1/1 -> Product3/1  "phimd"
  sum/1 -> Product1/2  "phimq"
  Mux1/1 -> phim_dq/1
  1/Ll_d/1 -> sum1/1
  phi/1 -> "phid phifd phikd "/1, phiq phikq1 (phikq2)/1
  phiq phikq1 (phikq2)/1 -> 1/Ll_q/1
  1/Ll_q/1 -> sum/1
  "phid phifd phikd "/1 -> 1/Ll_d/1
  Product3/1 -> Mux1/1  "phim_d"
  Product1/1 -> Mux1/2  "phim_q"

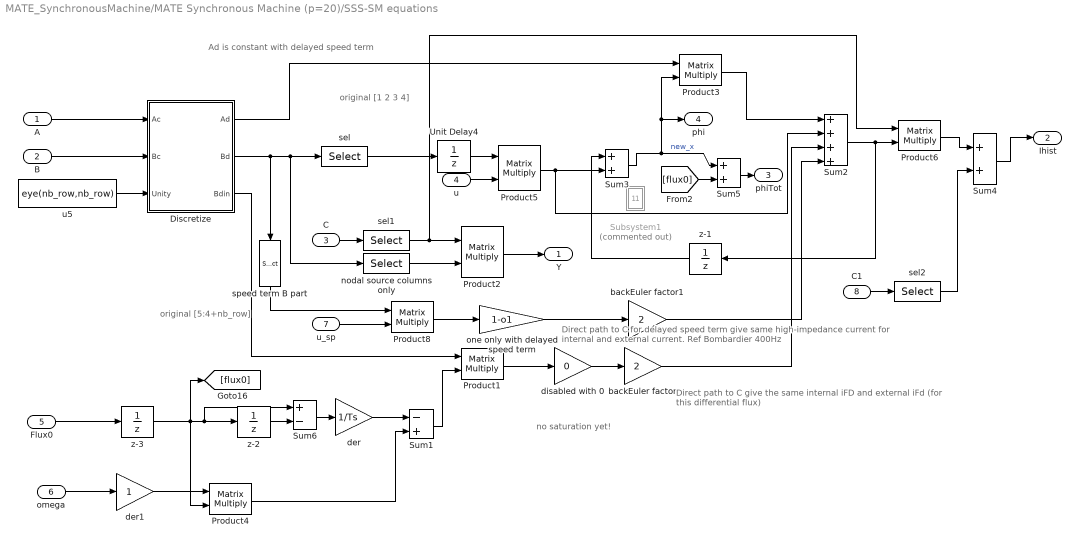
== system MATE_SynchronousMachine/MATE Synchronous Machine (p=20)/SSS-SM equations ==
  note: Direct path to C give the same internal iFD and external iFd
      | (for this differential flux)
  note: Direct path to C for delayed speed term give same high-impedance current
      | for internal and external current. Ref Bombardier 400Hz
  note: Ad is constant with delayed speed term
  note: original
      | [5:4+nb_row]
  note: original
      | [1 2 3  4]
  note: no saturation yet!
  A : Inport
  B : Inport  Port=2
  C : Inport  Port=3
  u : Inport  Port=4
  Flux0 : Inport  Port=5
  omega : Inport  Port=6
  u_sp : Inport  Port=7
  C1 : Inport  Port=8
  Discretize : Subsystem
  Product{1..6,8} (7 alike) : Product  Multiplication=Matrix(*)  SaturateOnIntegerOverflow=on  OutDataTypeStr=Inherit: Same as first input
  Subsystem1 : Subsystem  Commented=on
  Sum1 : Sum  Inputs=-+  SaturateOnIntegerOverflow=on
  Sum2 : Sum  Inputs=++++  SaturateOnIntegerOverflow=on
  Sum3 : Sum  SaturateOnIntegerOverflow=on
  Sum4 : Sum  Inputs=2  SaturateOnIntegerOverflow=on
  Sum5 : Sum  SaturateOnIntegerOverflow=on
  Sum6 : Sum  Inputs=+-  SaturateOnIntegerOverflow=on
  Unit Delay4 : UnitDelay  SampleTime=Ts  HasFrameUpgradeWarning=on
  backEuler factor : Gain  Gain=2  SaturateOnIntegerOverflow=on  OutDataTypeStr=Inherit: Same as input  ParamDataTypeStr=Inherit: Same as input
  backEuler factor1 : Gain  Gain=2  SaturateOnIntegerOverflow=on  OutDataTypeStr=Inherit: Same as input  ParamDataTypeStr=Inherit: Same as input
  der : Gain  Gain=1/Ts  SaturateOnIntegerOverflow=on  OutDataTypeStr=Inherit: Same as input  ParamDataTypeStr=Inherit: Same as input
  der1 : Gain  SaturateOnIntegerOverflow=on  OutDataTypeStr=Inherit: Same as input  ParamDataTypeStr=Inherit: Same as input
  disabled with 0 : Gain  Gain=0  SaturateOnIntegerOverflow=on  OutDataTypeStr=Inherit: Same as input  ParamDataTypeStr=Inherit: Same as input
  nodal source columns only : Selector  NumberOfDimensions=2  InputPortWidth=3  IndexOptions=Index vector (dialog),Index vector (dialog)  Indices=[1:nb_row],[1 2 3]  OutputSizes=1,1
  one only with delayed speed term : Gain  Gain=1-o1
  sel : Selector  NumberOfDimensions=2  InputPortWidth=3  IndexOptions=Index vector (dialog),Index vector (dialog)  Indices="[1:nb_row],[1 2 3  ]"  OutputSizes=1,1
  sel1 : Selector  NumberOfDimensions=2  InputPortWidth=3  IndexOptions=Index vector (dialog),Index vector (dialog)  Indices=[1 2 3 ],[1:nb_row]  OutputSizes=1,1
  sel2 : Selector  InputPortWidth=4  IndexOptions=Index vector (dialog)  Indices=[1 2 3 ]  OutputSizes=1
  speed term B part : Selector  NumberOfDimensions=2  InputPortWidth=3  IndexOptions=Index vector (dialog),Index vector (dialog)  Indices=[1:nb_row],[4:3+nb_row+1]  OutputSizes=1,1
  u5 : Constant  Value=eye(nb_row,nb_row)
  z-1 : UnitDelay  InitialCondition=flux_0  SampleTime=Ts  HasFrameUpgradeWarning=on
  z-2 : UnitDelay  SampleTime=Ts  HasFrameUpgradeWarning=on
  z-3 : UnitDelay  SampleTime=Ts  HasFrameUpgradeWarning=on
  Y : Outport
  Ihist : Outport  Port=2
  phiTot : Outport  Port=3
  phi : Outport  Port=4
  wires:
  disabled with 0/1 -> backEuler factor/1
  Product1/1 -> disabled with 0/1
  z-1/1 -> Sum3/1
  sel2/1 -> Sum4/2
  Sum4/1 -> Ihist/1
  Product6/1 -> Sum4/1
  C1/1 -> sel2/1
  sel1/1 -> Product2/1, Product6/1
  nodal source columns only/1 -> Product2/2
  u5/1 -> Discretize/3(Unity)
  Product2/1 -> Y/1
  A/1 -> Discretize/1(Ac)
  B/1 -> Discretize/2(Bc)
  C/1 -> sel1/1
  Product5/1 -> Sum2/2, Sum3/2
  Product3/1 -> Sum2/1
  Sum3/1 -> Sum5/1, phi/1, Product3/2  "new_x"
  Sum2/1 -> z-1/1, Product6/2
  Discretize/1(Ad) -> Product3/1
  u/1 -> Product5/2
  Discretize/2(Bd) -> nodal source columns only/1, sel/1, speed term B part/1
  Flux0/1 -> z-3/1
  Sum5/1 -> phiTot/1
  z-2/1 -> Sum6/2
  Sum6/1 -> der/1
  z-3/1 -> z-2/1, Sum6/1, [flux0], Product4/2
  Discretize/3(Bdin) -> Product1/1
  omega/1 -> der1/1
  Product4/1 -> Sum1/2
  der/1 -> Sum1/1
  [flux0] -> Sum5/2
  der1/1 -> Product4/1
  Sum1/1 -> Product1/2
  backEuler factor/1 -> Sum2/3
  Unit Delay4/1 -> Product5/1
  sel/1 -> Unit Delay4/1
  u_sp/1 -> Product8/2
  speed term B part/1 -> Product8/1
  Product8/1 -> one only with delayed speed term/1
  one only with delayed speed term/1 -> backEuler factor1/1
  backEuler factor1/1 -> Sum2/4

== system MATE_SynchronousMachine/MATE Synchronous Machine (p=20)/SSS-SM equations zero sequence only ==
  A : Inport
  B : Inport  Port=2
  C : Inport  Port=3
  u : Inport  Port=4
  Discretize : Subsystem
  Product{2..3,5..6} (4 alike) : Product  Multiplication=Matrix(*)  SaturateOnIntegerOverflow=on  OutDataTypeStr=Inherit: Same as first input
  Sum2 : Sum  SaturateOnIntegerOverflow=on
  Sum3 : Sum  SaturateOnIntegerOverflow=on
  u5 : Constant
  z-1 : UnitDelay  SampleTime=Ts  HasFrameUpgradeWarning=on
  Y0 : Outport
  Ihist0 : Outport  Port=2
  phi0 : Outport  Port=3
  wires:
  u5/1 -> Discretize/3(Unity)
  Product2/1 -> Y0/1
  A/1 -> Discretize/1(Ac)
  B/1 -> Discretize/2(Bc)
  C/1 -> Product6/1, Product2/1
  Product6/1 -> Ihist0/1
  Product5/1 -> Sum2/2, Sum3/2
  Product3/1 -> Sum2/1
  Sum3/1 -> Product3/2, phi0/1  "new_x"
  Sum2/1 -> z-1/1, Product6/2
  Discretize/1(Ad) -> Product3/1
  u/1 -> Product5/2
  z-1/1 -> Sum3/1
  Discretize/2(Bd) -> Product5/1, Product2/2
